simulink model "airspeed_controller"  (R2019b)
settings: Solver=VariableStepAuto  StartTime=0.0  StopTime=50  RelTol=1e-3
model workspace (MAT data in the model file):
  Cd = 0.5
  climb_max = 5
  g_common = 9.81
  mass_plane = 1.5
  nomThr = 0.3
  rou = 1.225
  sink_max = 1
  timeConstThrot = 8
libraries: simulink x1
settings Model: Creator=lee  LastModifiedBy=LEE
settings DataIOCC: ReturnWorkspaceOutputs=off
settings DebuggingCC: ArithmeticOperatorsInVariantConditions=warning
settings SFSimCC: CustomCodeUndefinedFunction=UseInterfaceOnly

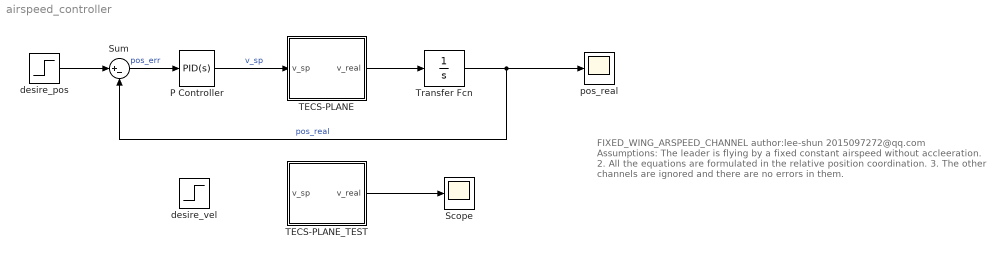
== system airspeed_controller ==
  note: FIXED_WING_ARSPEED_CHANNEL
      |
      | author:lee-shun 2015097272@qq.com
      |
      | Assumptions:
      |
      | The leader is flying by a fixed constant airspeed without accleeration.
      | 2. All the equations are formulated in the relative position coordination.
      | 3. The other channels are ignored and there are no errors in them.
  P Controller : simulink/Continuous/PID Controller  Controller=PID  Form=Parallel  TimeDomain=Continuous-time  SampleTime=-1  IntegratorMethod=Forward Euler  FilterMethod=Forward Euler  ControllerParametersSource=internal  P=0.2  I=0  D=0  UseFilter=on  N=100  TunerSelectOption=Transfer Function Based (PID Tuner App)  InitialConditionSource=internal  InitialConditionForIntegrator=0  InitialConditionForFilter=0  DifferentiatorICPrevScaledInput=0  ExternalReset=none  TrackingMode=off  Kt=1  LimitOutput=off  UpperSaturationLimit=inf  LowerSaturationLimit=-inf  LinearizeAsGain=on  AntiWindupMode=none  Kb=1  POutMin=[]  POutMax=[]  IOutMin=[]  IOutMax=[]  DOutMin=[]  DOutMax=[]  NOutMin=[]  NOutMax=[]  SumOutMin=[]  SumOutMax=[]  SaturationOutMin=[]  SaturationOutMax=[]  PParamMin=[]  PParamMax=[]  IParamMin=[]  IParamMax=[]  DParamMin=[]  DParamMax=[]  NParamMin=[]  NParamMax=[]  KbParamMin=[]  KbParamMax=[]  KtParamMin=[]  KtParamMax=[]  KbOutMin=[]  KbOutMax=[]  KtOutMin=[]  KtOutMax=[]  IntegratorOutMin=[]  IntegratorOutMax=[]  FilterOutMin=[]  FilterOutMax=[]  SumI1OutMin=[]  SumI1OutMax=[]  SumI2OutMin=[]  SumI2OutMax=[]  SumI3OutMin=[]  SumI3OutMax=[]  SumI4OutMin=[]  SumI4OutMax=[]  SumDOutMin=[]  SumDOutMax=[]  DifferentiatorOutMin=[]  DifferentiatorOutMax=[]  FilterDiffOutCoefMin=[]  FilterDiffOutCoefMax=[]  ReciprocalOutMin=[]  ReciprocalOutMax=[]  SumDenOutMin=[]  SumDenOutMax=[]  SumNumOutMin=[]  SumNumOutMax=[]  DivideOutMin=[]  DivideOutMax=[]  IntegratorContinuousStateAttributes=''  IntegratorStateMustResolveToSignalObject=off  IntegratorRTWStateStorageClass=Auto  FilterContinuousStateAttributes=''  FilterStateMustResolveToSignalObject=off  FilterRTWStateStorageClass=Auto  ParallelPVariant=InternalParameters  IdealPVariant=Disabled  IVariant=InternalParameters  DVariant=InternalParameters  IntegratorVariant=Continuous  SatVariant=Disabled  AWVariant=Passthrough  PCopyVariant=Disabled  TRVariant=Disabled  FdbkBlocksVariant=Forward  IdealPFdbkVariant=Disabled  SatFdbkVariant=Disabled  DerivativeFilterVariant=ContFilter  NVariant=InternalParameters  NCopyVariant=Disabled  FilterICVariant=InternalICsFilter  IntegratorICVariant=InternalICs  ExternalResetVariant=Disabled  TRSumVariant=Passthrough  SumFdbkVariant=Disabled  SumVariant=Sum_PID
  Scope : Scope
  Sum : Sum  Inputs=|+-
  TECS-PLANE : Subsystem
  TECS-PLANE_TEST : Subsystem
  Transfer Fcn : TransferFcn  Denominator=[1 0]
  desire_pos : Step  After=5  SampleTime=0
  desire_vel : Step  After=0  SampleTime=0
  pos_real : Scope
  wires:
  Sum/1 -> P Controller/1  "pos_err"
  Transfer Fcn/1 -> pos_real/1, Sum/2  "pos_real"
  desire_pos/1 -> Sum/1
  P Controller/1 -> TECS-PLANE/1(v_sp)  "v_sp"
  TECS-PLANE/1(v_real) -> Transfer Fcn/1
  TECS-PLANE_TEST/1(v_real) -> Scope/1

== system airspeed_controller/TECS-PLANE ==
  v_sp : Inport
  PLANE : Subsystem
  Saturation : Saturate  UpperLimit=1  LowerLimit=0
  "TECS " : Subsystem
  v_real : Outport
  wires:
  PLANE/1(v_real) -> v_real/1, "TECS "/2(v_real)  "v_real"
  Saturation/1 -> PLANE/1(thrust)  "limited_tr"
  "TECS "/1(thrust) -> Saturation/1  "thrust"
  v_sp/1 -> "TECS "/1(v_sp)

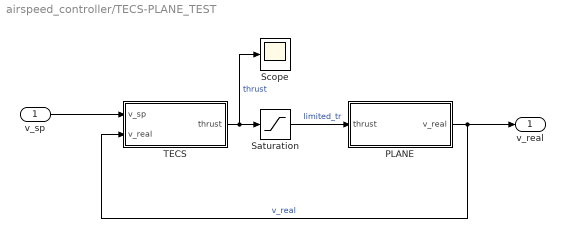
== system airspeed_controller/TECS-PLANE_TEST ==
  v_sp : Inport
  PLANE : Subsystem
  Saturation : Saturate  UpperLimit=1  LowerLimit=0
  Scope : Scope
  "TECS " : Subsystem
  v_real : Outport
  wires:
  PLANE/1(v_real) -> v_real/1, "TECS "/2(v_real)  "v_real"
  Saturation/1 -> PLANE/1(thrust)  "limited_tr"
  "TECS "/1(thrust) -> Scope/1, Saturation/1  "thrust"
  v_sp/1 -> "TECS "/1(v_sp)

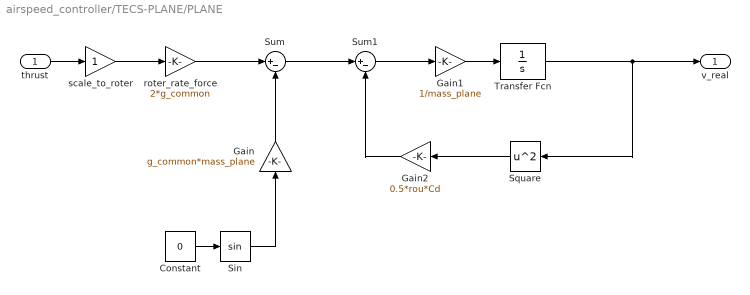
== system airspeed_controller/TECS-PLANE/PLANE ==
  thrust : Inport
  Constant : Constant  Value=0
  Gain : Gain  Gain=g_common*mass_plane
  Gain1 : Gain  Gain=1/mass_plane
  Gain2 : Gain  Gain=0.5*rou*Cd
  Sin : Trigonometry
  Square : Math  Operator=square  SignedPower=off  SaturateOnIntegerOverflow=on
  Sum : Sum  Inputs=|+-
  Sum1 : Sum  Inputs=|+-
  Transfer Fcn : TransferFcn  Denominator=[1 0]
  roter_rate_force : Gain  Gain=2*g_common
  scale_to_roter : Gain
  v_real : Outport
  wires:
  thrust/1 -> scale_to_roter/1
  scale_to_roter/1 -> roter_rate_force/1
  roter_rate_force/1 -> Sum/1
  Gain/1 -> Sum/2
  Constant/1 -> Sin/1
  Sin/1 -> Gain/1
  Sum/1 -> Sum1/1
  Sum1/1 -> Gain1/1
  Gain1/1 -> Transfer Fcn/1
  Transfer Fcn/1 -> Square/1, v_real/1
  Square/1 -> Gain2/1
  Gain2/1 -> Sum1/2

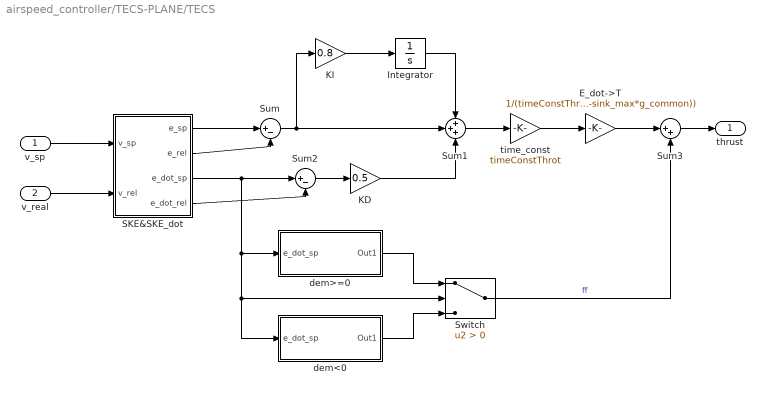
== system airspeed_controller/TECS-PLANE/TECS  ==
  v_sp : Inport
  v_real : Inport  Port=2
  E_dot->T : Gain  Gain=1/(timeConstThrot*(climb_max*g_common-sink_max*g_common))
  Integrator : Integrator
  KD : Gain  Gain=0.5
  KI : Gain  Gain=0.8
  SKE&SKE_dot : Subsystem
  Sum : Sum  Inputs=|+-
  Sum1 : Sum  Inputs=+++
  Sum2 : Sum  Inputs=|+-
  Sum3 : Sum  Inputs=|++
  Switch : Switch  Criteria=u2 > Threshold
  dem<0 : Subsystem
  dem>=0 : Subsystem
  time_const : Gain  Gain=timeConstThrot
  thrust : Outport
  wires:
  Sum/1 -> Sum1/2, KI/1
  KI/1 -> Integrator/1
  Integrator/1 -> Sum1/1
  Sum1/1 -> time_const/1
  time_const/1 -> E_dot->T/1
  E_dot->T/1 -> Sum3/1
  v_sp/1 -> SKE&SKE_dot/1(v_sp)
  v_real/1 -> SKE&SKE_dot/2(v_rel)
  SKE&SKE_dot/1(e_sp) -> Sum/1
  SKE&SKE_dot/2(e_rel) -> Sum/2
  SKE&SKE_dot/3(e_dot_sp) -> dem<0/1(e_dot_sp), Switch/2, dem>=0/1(e_dot_sp), Sum2/1
  SKE&SKE_dot/4(e_dot_rel) -> Sum2/2
  Sum2/1 -> KD/1
  KD/1 -> Sum1/3
  Sum3/1 -> thrust/1
  Switch/1 -> Sum3/2  "ff"
  dem>=0/1(Out1) -> Switch/1
  dem<0/1(Out1) -> Switch/3

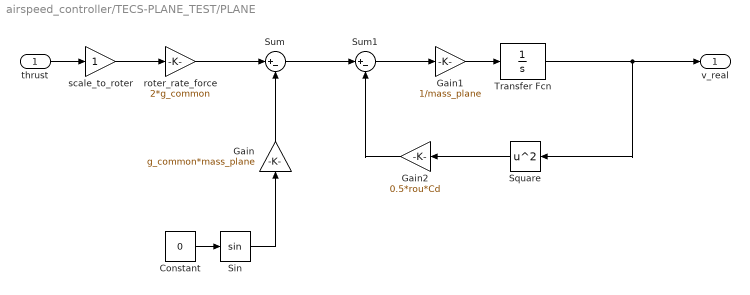
== system airspeed_controller/TECS-PLANE_TEST/PLANE ==
  thrust : Inport
  Constant : Constant  Value=0
  Gain : Gain  Gain=g_common*mass_plane
  Gain1 : Gain  Gain=1/mass_plane
  Gain2 : Gain  Gain=0.5*rou*Cd
  Sin : Trigonometry
  Square : Math  Operator=square  SignedPower=off  SaturateOnIntegerOverflow=on
  Sum : Sum  Inputs=|+-
  Sum1 : Sum  Inputs=|+-
  Transfer Fcn : TransferFcn  Denominator=[1 0]
  roter_rate_force : Gain  Gain=2*g_common
  scale_to_roter : Gain
  v_real : Outport
  wires:
  thrust/1 -> scale_to_roter/1
  scale_to_roter/1 -> roter_rate_force/1
  roter_rate_force/1 -> Sum/1
  Gain/1 -> Sum/2
  Constant/1 -> Sin/1
  Sin/1 -> Gain/1
  Sum/1 -> Sum1/1
  Sum1/1 -> Gain1/1
  Gain1/1 -> Transfer Fcn/1
  Transfer Fcn/1 -> Square/1, v_real/1
  Square/1 -> Gain2/1
  Gain2/1 -> Sum1/2

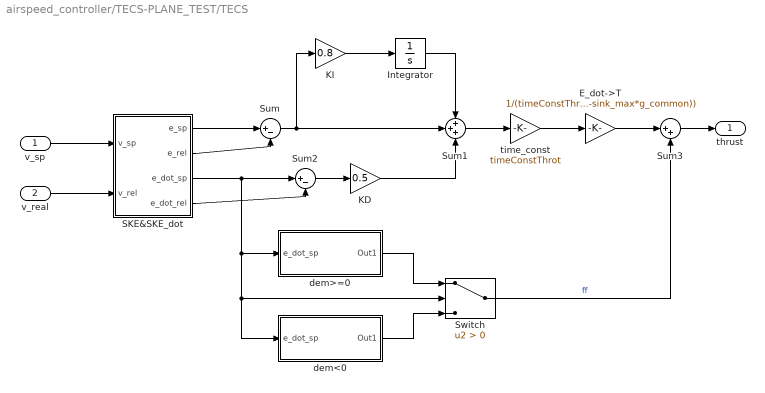
== system airspeed_controller/TECS-PLANE_TEST/TECS  ==
  v_sp : Inport
  v_real : Inport  Port=2
  E_dot->T : Gain  Gain=1/(timeConstThrot*(climb_max*g_common-sink_max*g_common))
  Integrator : Integrator
  KD : Gain  Gain=0.5
  KI : Gain  Gain=0.8
  SKE&SKE_dot : Subsystem
  Sum : Sum  Inputs=|+-
  Sum1 : Sum  Inputs=+++
  Sum2 : Sum  Inputs=|+-
  Sum3 : Sum  Inputs=|++
  Switch : Switch  Criteria=u2 > Threshold
  dem<0 : Subsystem
  dem>=0 : Subsystem
  time_const : Gain  Gain=timeConstThrot
  thrust : Outport
  wires:
  Sum/1 -> Sum1/2, KI/1
  KI/1 -> Integrator/1
  Integrator/1 -> Sum1/1
  Sum1/1 -> time_const/1
  time_const/1 -> E_dot->T/1
  E_dot->T/1 -> Sum3/1
  v_sp/1 -> SKE&SKE_dot/1(v_sp)
  v_real/1 -> SKE&SKE_dot/2(v_rel)
  SKE&SKE_dot/1(e_sp) -> Sum/1
  SKE&SKE_dot/2(e_rel) -> Sum/2
  SKE&SKE_dot/3(e_dot_sp) -> dem<0/1(e_dot_sp), Switch/2, dem>=0/1(e_dot_sp), Sum2/1
  SKE&SKE_dot/4(e_dot_rel) -> Sum2/2
  Sum2/1 -> KD/1
  KD/1 -> Sum1/3
  Sum3/1 -> thrust/1
  Switch/1 -> Sum3/2  "ff"
  dem>=0/1(Out1) -> Switch/1
  dem<0/1(Out1) -> Switch/3

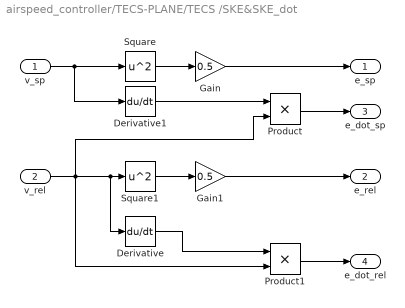
== system airspeed_controller/TECS-PLANE/TECS /SKE&SKE_dot ==
  v_sp : Inport
  v_rel : Inport  Port=2
  Derivative : Derivative
  Derivative1 : Derivative
  Gain : Gain  Gain=0.5
  Gain1 : Gain  Gain=0.5
  Product : Product
  Product1 : Product
  Square : Math  Operator=square  SignedPower=off  SaturateOnIntegerOverflow=on
  Square1 : Math  Operator=square  SignedPower=off  SaturateOnIntegerOverflow=on
  e_sp : Outport
  e_rel : Outport  Port=2
  e_dot_sp : Outport  Port=3
  e_dot_rel : Outport  Port=4
  wires:
  Square/1 -> Gain/1
  Square1/1 -> Gain1/1
  Gain/1 -> e_sp/1
  v_sp/1 -> Derivative1/1, Square/1
  Gain1/1 -> e_rel/1
  Product/1 -> e_dot_sp/1
  v_rel/1 -> Product1/2, Product/2, Derivative/1, Square1/1
  Product1/1 -> e_dot_rel/1
  Derivative1/1 -> Product/1
  Derivative/1 -> Product1/1

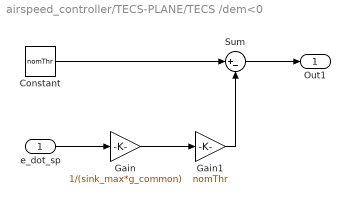
== system airspeed_controller/TECS-PLANE/TECS /dem<0 ==
  e_dot_sp : Inport
  Constant : Constant  Value=nomThr
  Gain : Gain  Gain=1/(sink_max*g_common)
  Gain1 : Gain  Gain=nomThr
  Sum : Sum  Inputs=|+-
  Out1 : Outport
  wires:
  Constant/1 -> Sum/1
  e_dot_sp/1 -> Gain/1
  Gain/1 -> Gain1/1
  Gain1/1 -> Sum/2
  Sum/1 -> Out1/1

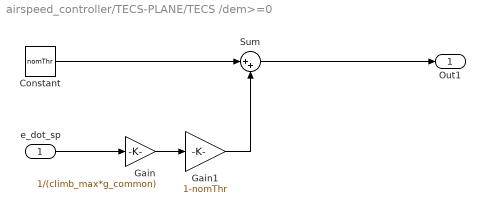
== system airspeed_controller/TECS-PLANE/TECS /dem>=0 ==
  e_dot_sp : Inport
  Constant : Constant  Value=nomThr
  Gain : Gain  Gain=1/(climb_max*g_common)
  Gain1 : Gain  Gain=1-nomThr
  Sum : Sum  Inputs=|++
  Out1 : Outport
  wires:
  Constant/1 -> Sum/1
  e_dot_sp/1 -> Gain/1
  Gain/1 -> Gain1/1
  Gain1/1 -> Sum/2
  Sum/1 -> Out1/1

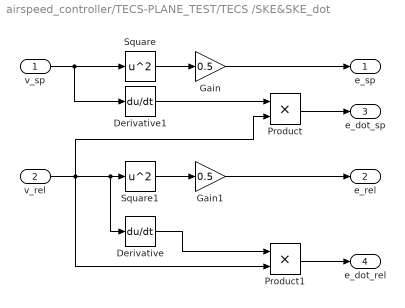
== system airspeed_controller/TECS-PLANE_TEST/TECS /SKE&SKE_dot ==
  v_sp : Inport
  v_rel : Inport  Port=2
  Derivative : Derivative
  Derivative1 : Derivative
  Gain : Gain  Gain=0.5
  Gain1 : Gain  Gain=0.5
  Product : Product
  Product1 : Product
  Square : Math  Operator=square  SignedPower=off  SaturateOnIntegerOverflow=on
  Square1 : Math  Operator=square  SignedPower=off  SaturateOnIntegerOverflow=on
  e_sp : Outport
  e_rel : Outport  Port=2
  e_dot_sp : Outport  Port=3
  e_dot_rel : Outport  Port=4
  wires:
  Square/1 -> Gain/1
  Square1/1 -> Gain1/1
  Gain/1 -> e_sp/1
  v_sp/1 -> Derivative1/1, Square/1
  Gain1/1 -> e_rel/1
  Product/1 -> e_dot_sp/1
  v_rel/1 -> Product1/2, Product/2, Derivative/1, Square1/1
  Product1/1 -> e_dot_rel/1
  Derivative1/1 -> Product/1
  Derivative/1 -> Product1/1

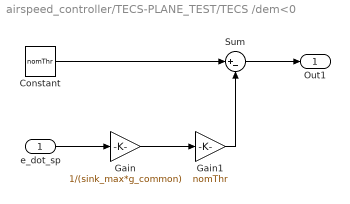
== system airspeed_controller/TECS-PLANE_TEST/TECS /dem<0 ==
  e_dot_sp : Inport
  Constant : Constant  Value=nomThr
  Gain : Gain  Gain=1/(sink_max*g_common)
  Gain1 : Gain  Gain=nomThr
  Sum : Sum  Inputs=|+-
  Out1 : Outport
  wires:
  Constant/1 -> Sum/1
  e_dot_sp/1 -> Gain/1
  Gain/1 -> Gain1/1
  Gain1/1 -> Sum/2
  Sum/1 -> Out1/1

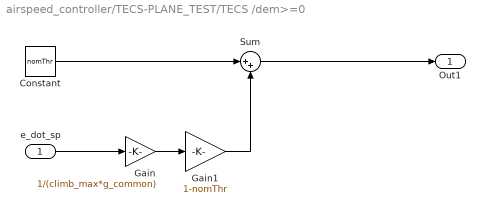
== system airspeed_controller/TECS-PLANE_TEST/TECS /dem>=0 ==
  e_dot_sp : Inport
  Constant : Constant  Value=nomThr
  Gain : Gain  Gain=1/(climb_max*g_common)
  Gain1 : Gain  Gain=1-nomThr
  Sum : Sum  Inputs=|++
  Out1 : Outport
  wires:
  Constant/1 -> Sum/1
  e_dot_sp/1 -> Gain/1
  Gain/1 -> Gain1/1
  Gain1/1 -> Sum/2
  Sum/1 -> Out1/1
